simulink model "RealSpace_Pheromone_Model_old"  (R2025b)
settings: Solver=ode4  StartTime=0  StopTime=60  FixedStep=0.01  RelTol=1e-3
undefined symbols (not defined in the file or in its folder): DiscIntNeverNeededParam
libraries: slpidlib x1
settings Model: Creator=chandansheikder  LastModifiedBy=chandansheikder
settings DataIOCC: SaveFormat=Array

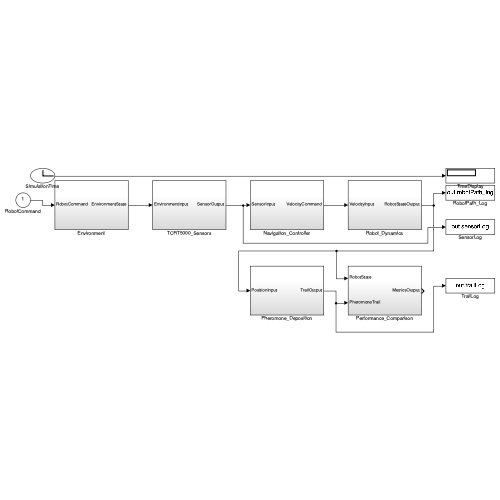
[thumbnail: Simulink's stored preview of the top-level diagram]
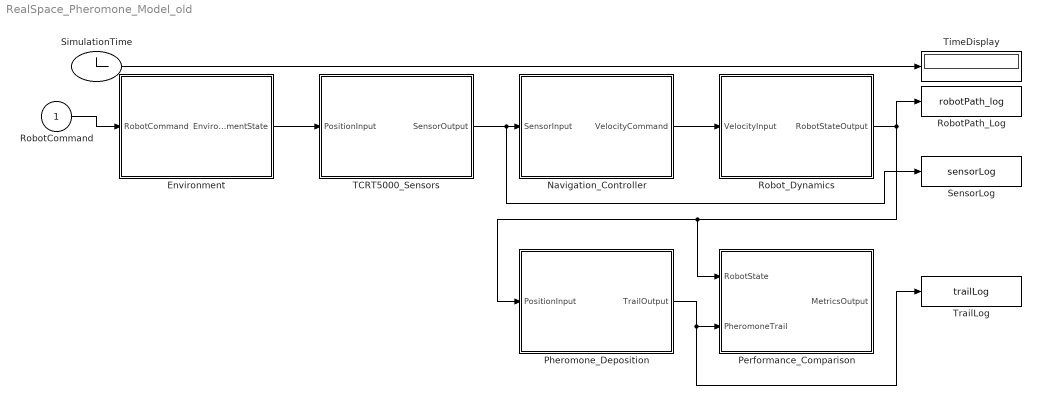
== system RealSpace_Pheromone_Model_old ==
  RobotCommand : Inport
  Environment : Subsystem
  Navigation_Controller : Subsystem
  Performance_Comparison : Subsystem
  Pheromone_Deposition : Subsystem
  RobotPath_Log : ToWorkspace  VariableName=robotPath_log  SaveFormat=Timeseries  SampleTime=0.1
  Robot_Dynamics : Subsystem
  SensorLog : ToWorkspace  VariableName=sensorLog  SaveFormat=Timeseries  SampleTime=0.1
  SimulationTime : Clock
  TCRT5000_Sensors : Subsystem
  TimeDisplay : Display
  TrailLog : ToWorkspace  VariableName=trailLog  SaveFormat=Timeseries  SampleTime=0.5
  wires:
  Environment/1(EnvironmentState) -> TCRT5000_Sensors/1(PositionInput)
  Navigation_Controller/1(VelocityCommand) -> Robot_Dynamics/1(VelocityInput)
  TCRT5000_Sensors/1(SensorOutput) -> SensorLog/1, Navigation_Controller/1(SensorInput)
  Robot_Dynamics/1(RobotStateOutput) -> Pheromone_Deposition/1(PositionInput), Performance_Comparison/1(RobotState), RobotPath_Log/1
  Pheromone_Deposition/1(TrailOutput) -> TrailLog/1, Performance_Comparison/2(PheromoneTrail)
  SimulationTime/1 -> TimeDisplay/1
  RobotCommand/1 -> Environment/1(RobotCommand)

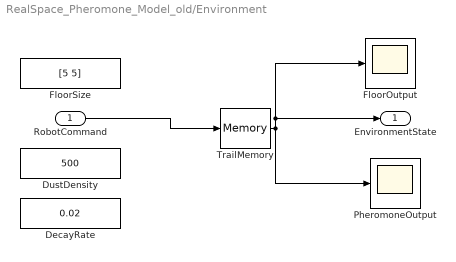
== system RealSpace_Pheromone_Model_old/Environment ==
  RobotCommand : Inport
  DecayRate : Constant  Value=0.02
  DustDensity : Constant  Value=500
  FloorOutput : Scope
  FloorSize : Constant  Value=[5 5]
  PheromoneOutput : Scope
  TrailMemory : Memory  InitialCondition=[0 0 0]
  EnvironmentState : Outport
  wires:
  RobotCommand/1 -> TrailMemory/1
  TrailMemory/1 -> PheromoneOutput/1, FloorOutput/1, EnvironmentState/1

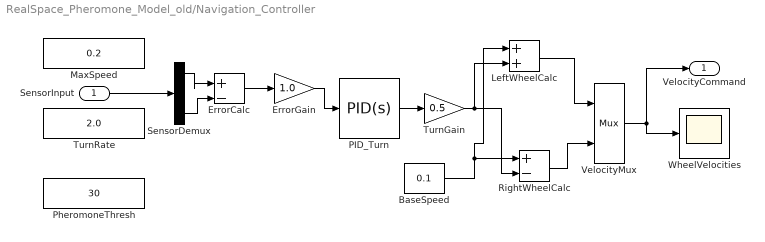
== system RealSpace_Pheromone_Model_old/Navigation_Controller ==
  SensorInput : Inport
  BaseSpeed : Constant  Value=0.1
  ErrorCalc : Sum  Inputs=|+-
  ErrorGain : Gain  Gain=1.0
  LeftWheelCalc : Sum
  MaxSpeed : Constant  Value=0.2
  PID_Turn : slpidlib/PID Controller  Controller=PID  Form=Parallel  TimeDomain=Continuous-time  UseExternalTs=off  SampleTime=-1  IntegratorMethod=Forward Euler  FilterMethod=Forward Euler  ControllerParametersSource=internal  P=3.0  I=0.1  UseKiTs=off  D=0.5  UseExternalDerivativeSource=off  N=100  UseFilter=on  TunerSelectOption=Transfer Function Based (PID Tuner App)  InitialConditionSource=internal  InitialConditionForIntegrator=0  InitialConditionForFilter=0  DifferentiatorICPrevScaledInput=0  ExternalReset=none  TrackingMode=off  Kt=1  LimitOutput=off  SatLimitsSource=internal  UpperSaturationLimit=inf  LowerSaturationLimit=-inf  LinearizeAsGain=on  AntiWindupMode=none  Kb=1  LimitIntegrator=off  UpperIntegratorSaturationLimit=inf  LowerIntegratorSaturationLimit=-inf  POutMin=[]  POutMax=[]  IOutMin=[]  IOutMax=[]  DOutMin=[]  DOutMax=[]  NOutMin=[]  NOutMax=[]  SumOutMin=[]  SumOutMax=[]  SaturationOutMin=[]  SaturationOutMax=[]  PParamMin=[]  PParamMax=[]  IParamMin=[]  IParamMax=[]  DParamMin=[]  DParamMax=[]  NParamMin=[]  NParamMax=[]  KbParamMin=[]  KbParamMax=[]  KtParamMin=[]  KtParamMax=[]  KbOutMin=[]  KbOutMax=[]  KtOutMin=[]  KtOutMax=[]  IntegratorOutMin=[]  IntegratorOutMax=[]  FilterOutMin=[]  FilterOutMax=[]  SumI1OutMin=[]  SumI1OutMax=[]  SumI2OutMin=[]  SumI2OutMax=[]  SumI3OutMin=[]  SumI3OutMax=[]  SumI4OutMin=[]  SumI4OutMax=[]  SumDOutMin=[]  SumDOutMax=[]  DifferentiatorOutMin=[]  DifferentiatorOutMax=[]  FilterDiffOutCoefMin=[]  FilterDiffOutCoefMax=[]  ReciprocalOutMin=[]  ReciprocalOutMax=[]  SumDenOutMin=[]  SumDenOutMax=[]  SumNumOutMin=[]  SumNumOutMax=[]  DivideOutMin=[]  DivideOutMax=[]  UdiffTsProdOutMin=[]  UdiffTsProdOutMax=[]  NTsProdOutMin=[]  NTsProdOutMax=[]  UintegralTsProdOutMin=[]  UintegralTsProdOutMax=[]  UngainTsProdOutMin=[]  UngainTsProdOutMax=[]  ClampingZeroOutDataTypeStr=Inherit: Inherit via back propagation  ClampingZeroOutMin=[]  ClampingZeroOutMax=[]  FilterDenConstantOutDataTypeStr=Inherit: Inherit via back propagation  FilterDenConstantOutMin=[]  FilterDenConstantOutMax=[]  PCopyOutDataTypeStr=Inherit: Inherit via back propagation  PCopyOutMin=[]  PCopyOutMax=[]  NCopyOutDataTypeStr=Inherit: Inherit via back propagation  NCopyOutMin=[]  NCopyOutMax=[]  IntegratorContinuousStateAttributes=''  IntegratorStateMustResolveToSignalObject=off  IntegratorRTWStateStorageClass=Auto  FilterContinuousStateAttributes=''  FilterStateMustResolveToSignalObject=off  FilterRTWStateStorageClass=Auto  ParallelPVariant=InternalParameters  IdealPVariant=Disabled  IVariant=InternalParameters  DVariant=InternalParameters  IntegratorVariant=Continuous  SatVariant=Disabled  AWVariant=Passthrough  PCopyVariant=Disabled  TRVariant=Disabled  FdbkBlocksVariant=Forward  IdealPFdbkVariant=Disabled  SatFdbkVariant=Disabled  DerivativeFilterVariant=ContFilter  NVariant=InternalParameters  NCopyVariant=Disabled  FilterICVariant=InternalICsFilter  IntegratorICVariant=InternalICs  ExternalResetVariant=Disabled  TRSumVariant=Passthrough  SumFdbkVariant=Disabled  SumVariant=Sum_PID  TsampFilterVariant=InternalTs  TsampNgainVariant=Passthrough  TsampIntegralVariant=Disabled_SignalSpec  ExternalSaturationOutDataTypeStr=Inherit: Same as second input  DerivativeSourceVariant=ErrorSignal  PreIntVariant=InternalPreInt
  PheromoneThresh : Constant  Value=30
  RightWheelCalc : Sum  Inputs=+-
  SensorDemux : Demux  Outputs=3
  TurnGain : Gain  Gain=0.5
  TurnRate : Constant  Value=2.0
  VelocityMux : Mux  Inputs=2
  WheelVelocities : Scope
  VelocityCommand : Outport
  wires:
  SensorInput/1 -> SensorDemux/1
  SensorDemux/1 -> ErrorCalc/1
  SensorDemux/3 -> ErrorCalc/2
  ErrorCalc/1 -> ErrorGain/1
  ErrorGain/1 -> PID_Turn/1
  PID_Turn/1 -> TurnGain/1
  TurnGain/1 -> LeftWheelCalc/2, RightWheelCalc/2
  BaseSpeed/1 -> LeftWheelCalc/1, RightWheelCalc/1
  LeftWheelCalc/1 -> VelocityMux/1
  RightWheelCalc/1 -> VelocityMux/2
  VelocityMux/1 -> VelocityCommand/1, WheelVelocities/1

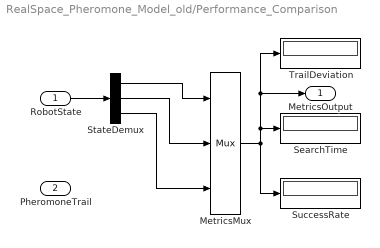
== system RealSpace_Pheromone_Model_old/Performance_Comparison ==
  RobotState : Inport
  PheromoneTrail : Inport  Port=2
  MetricsMux : Mux  Inputs=3
  SearchTime : Display
  StateDemux : Demux  Outputs=3
  SuccessRate : Display
  TrailDeviation : Display
  MetricsOutput : Outport
  wires:
  RobotState/1 -> StateDemux/1
  StateDemux/1 -> MetricsMux/1
  StateDemux/2 -> MetricsMux/2
  StateDemux/3 -> MetricsMux/3
  MetricsMux/1 -> TrailDeviation/1, MetricsOutput/1, SearchTime/1, SuccessRate/1

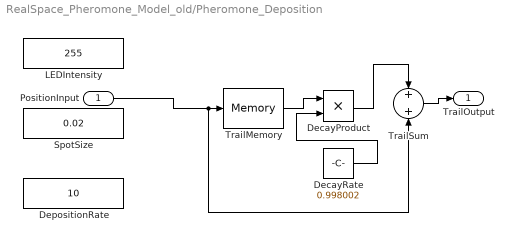
== system RealSpace_Pheromone_Model_old/Pheromone_Deposition ==
  PositionInput : Inport
  DecayProduct : Product
  DecayRate : Constant  Value=0.998002
  DepositionRate : Constant  Value=10
  LEDIntensity : Constant  Value=255
  SpotSize : Constant  Value=0.02
  TrailMemory : Memory  InitialCondition=[0 0 0]
  TrailSum : Sum
  TrailOutput : Outport
  wires:
  DecayRate/1 -> DecayProduct/2
  PositionInput/1 -> TrailSum/2, TrailMemory/1
  DecayProduct/1 -> TrailSum/1
  TrailMemory/1 -> DecayProduct/1
  TrailSum/1 -> TrailOutput/1

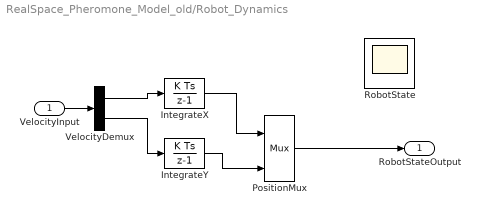
== system RealSpace_Pheromone_Model_old/Robot_Dynamics ==
  VelocityInput : Inport
  IntegrateX : DiscreteIntegrator  ICPrevOutput=DiscIntNeverNeededParam  ICPrevScaledInput=DiscIntNeverNeededParam
  IntegrateY : DiscreteIntegrator  ICPrevOutput=DiscIntNeverNeededParam  ICPrevScaledInput=DiscIntNeverNeededParam
  PositionMux : Mux  Inputs=2
  RobotState : Scope
  VelocityDemux : Demux  Outputs=2
  RobotStateOutput : Outport
  wires:
  VelocityInput/1 -> VelocityDemux/1
  VelocityDemux/1 -> IntegrateX/1
  VelocityDemux/2 -> IntegrateY/1
  IntegrateX/1 -> PositionMux/1
  IntegrateY/1 -> PositionMux/2
  PositionMux/1 -> RobotStateOutput/1

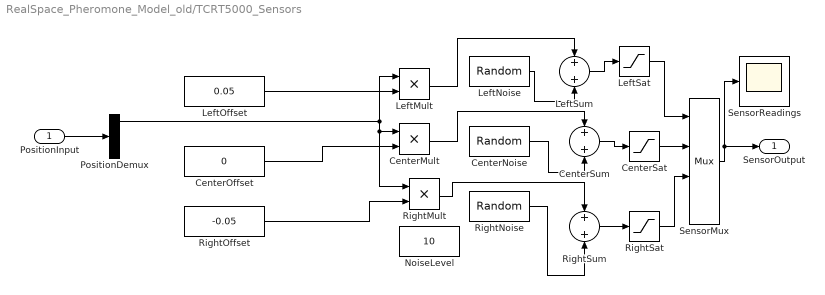
== system RealSpace_Pheromone_Model_old/TCRT5000_Sensors ==
  PositionInput : Inport
  CenterMult : Product
  CenterNoise : RandomNumber  Variance=100
  CenterOffset : Constant  Value=0
  CenterSat : Saturation  LowerLimit=0  UpperLimit=255
  CenterSum : Sum
  LeftMult : Product
  LeftNoise : RandomNumber  Variance=100
  LeftOffset : Constant  Value=0.05
  LeftSat : Saturation  LowerLimit=0  UpperLimit=255
  LeftSum : Sum
  NoiseLevel : Constant  Value=10
  PositionDemux : Demux  Outputs=2
  RightMult : Product
  RightNoise : RandomNumber  Variance=100
  RightOffset : Constant  Value=-0.05
  RightSat : Saturation  LowerLimit=0  UpperLimit=255
  RightSum : Sum
  SensorMux : Mux  Inputs=3
  SensorReadings : Scope
  SensorOutput : Outport
  wires:
  PositionInput/1 -> PositionDemux/1
  PositionDemux/1 -> RightMult/1, CenterMult/1, LeftMult/1
  LeftOffset/1 -> LeftMult/2
  CenterOffset/1 -> CenterMult/2
  RightOffset/1 -> RightMult/2
  LeftMult/1 -> LeftSum/1
  CenterMult/1 -> CenterSum/1
  RightMult/1 -> RightSum/1
  LeftNoise/1 -> LeftSum/2
  CenterNoise/1 -> CenterSum/2
  RightNoise/1 -> RightSum/2
  LeftSum/1 -> LeftSat/1
  CenterSum/1 -> CenterSat/1
  RightSum/1 -> RightSat/1
  LeftSat/1 -> SensorMux/1
  CenterSat/1 -> SensorMux/2
  RightSat/1 -> SensorMux/3
  SensorMux/1 -> SensorReadings/1, SensorOutput/1
